simulink model "RLS"  (R2022b)
settings: Solver=FixedStepAuto  StartTime=0.0  StopTime=10  FixedStep=0.001  RelTol=1e-3
libraries: simulink x1
settings Model: Creator=artur  LastModifiedBy=artur

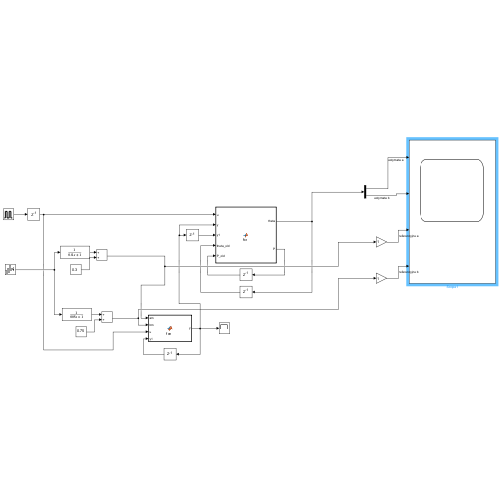
[thumbnail: Simulink's stored preview of the top-level diagram]
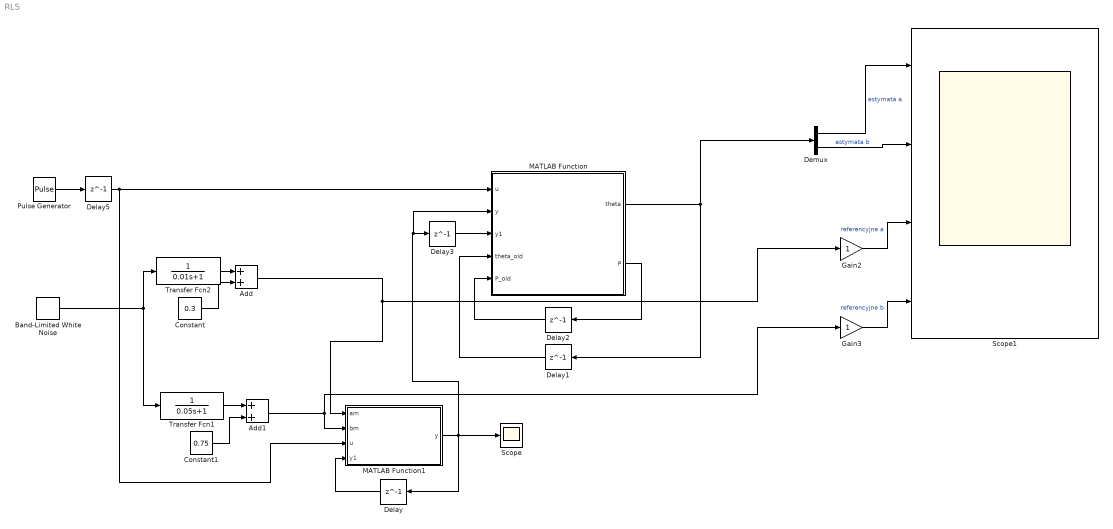
== system RLS ==
  Add : Sum
  Add1 : Sum
  Band-Limited White Noise : simulink/Sources/Band-Limited White Noise  Cov=[0.0001]  Ts=0.3  seed=[13524123]  VectorParams1D=off
  Constant : Constant  Value=0.3
  Constant1 : Constant  Value=0.75
  Delay : Delay  DelayLength=1  InitialCondition=0
  Delay1 : Delay  DelayLength=1  InitialCondition=[0.25 0.65]
  Delay2 : Delay  DelayLength=1  InitialCondition=eye(2)*10^6
  Delay3 : Delay  DelayLength=1  InitialCondition=0
  Delay5 : Delay  DelayLength=1  InitialCondition=0
  Demux : Demux  Outputs=2
  Gain2 : Gain
  Gain3 : Gain
  MATLAB Function : MATLAB Function  TreatAsAtomicUnit=on
  MATLAB Function1 : MATLAB Function  TreatAsAtomicUnit=on
  Pulse Generator : DiscretePulseGenerator  PulseType=Time based  Period=0.1  PulseWidth=50
  Scope : Scope
  Scope1 : Scope  NumInputPorts=4
  Transfer Fcn1 : TransferFcn  Denominator=[0.05 1]
  Transfer Fcn2 : TransferFcn  Denominator=[0.01 1]
  wires:
  MATLAB Function1/1(y) -> MATLAB Function/2(y), Delay3/1, Delay/1, Scope/1
  Delay/1 -> MATLAB Function1/4(y1)
  MATLAB Function/1(theta) -> Demux/1, Delay1/1
  Delay1/1 -> MATLAB Function/4(theta_old)
  MATLAB Function/2(P) -> Delay2/1
  Delay2/1 -> MATLAB Function/5(P_old)
  Delay3/1 -> MATLAB Function/3(y1)
  Delay5/1 -> MATLAB Function/1(u), MATLAB Function1/3(u)
  Pulse Generator/1 -> Delay5/1
  Demux/1 -> Scope1/1  "estymata a"
  Demux/2 -> Scope1/2  "estymata b"
  Gain2/1 -> Scope1/3  "referencyjne a"
  Gain3/1 -> Scope1/4  "referencyjne b"
  Constant/1 -> Add/2
  Constant1/1 -> Add1/2
  Band-Limited White Noise/1 -> Transfer Fcn2/1, Transfer Fcn1/1
  Add/1 -> MATLAB Function1/1(am), Gain2/1
  Add1/1 -> MATLAB Function1/2(bm), Gain3/1
  Transfer Fcn2/1 -> Add/1
  Transfer Fcn1/1 -> Add1/1

== matlab function RLS/MATLAB Function ==
  data: u input; theta output; y input; y1 input; theta_old input; P_old input; P output
function [theta,P] = fcn(u,y,y1,theta_old,P_old)

phi = [y1;u];
lambda = 0.97;

K = P_old * phi * 1/(lambda + phi'*P_old*phi);

P = 1/lambda * (eye(2) - K*phi') * P_old;

theta = theta_old + K * (y - phi'*theta_old);

== matlab function RLS/MATLAB Function1 ==
  data: am input; bm input; u input; y1 input; y output
function y = fcn(am,bm,u,y1)

y = am * y1 + bm * u;
